simulink model "qless_forgetting_factor_16x16_nofifo"  (R2021a)
settings: Solver=FixedStepDiscrete  StartTime=0.0  StopTime=stoptime*inf  RelTol=1e-3
InitFcn:
  | qless_init_16chan_fi
undefined symbols (not defined in the file): fc, numArrayElements, physconst, srcAngles, Ts
libraries: hdlsllib x137, commfilt2 x4, commrfcorlib x3, commsync2 x3, commrflib2 x2, commrandsrc3 x2, simulink x2, phasedtxrxlib x2, commdigbbndcpm2 x1, embreciprocals x1, commdigbbndpm3 x1
(part 1 of 22)
Description:
  | MVDR HDL 4x4 systolic testbench
settings Model: DataTypeOverride=Off  SimulationMode=accelerator  Creator=The MathWorks, Inc.  LastModifiedBy=darenlee
settings SolverCC: AlgebraicLoopSolver=TrustRegion
settings DataIOCC: LimitDataPoints=on  SaveFormat=Array  SaveOutput=off  SaveTime=off  ReturnWorkspaceOutputs=off
settings OptimizationCC: BlockReduction=off  ConditionallyExecuteInputs=off  DefaultParameterBehavior=Inlined  LifeSpan=inf
settings DebuggingCC: ReadBeforeWriteMsg=DisableAll  WriteAfterWriteMsg=DisableAll  WriteAfterReadMsg=DisableAll  AlgebraicLoopMsg=error  UnderspecifiedInitializationDetection=Classic  MergeDetectMultiDrivingBlocksExec=none  SolverPrmCheckMsg=warning  SingleTaskRateTransMsg=error  ParameterPrecisionLossMsg=none  AllowSymbolicDim=off  SFUnexpectedBacktrackingDiag=warning  SFNoUnconditionalDefaultTransitionDiag=warning  SFExecutionAtInitializationDiag=none  SFMachineParentedDataDiag=warning  ArithmeticOperatorsInVariantConditions=warning
settings HardwareCC: ProdBitPerPointer=32  ProdBitPerSizeT=32  ProdBitPerPtrDiffT=32  ProdLargestAtomicFloat=None  ProdIntDivRoundTo=Undefined  ProdEndianess=Unspecified  ProdWordSize=32  ProdHWDeviceType=ASIC/FPGA->ASIC/FPGA  TargetBitPerPointer=64  TargetBitPerSizeT=64  TargetBitPerPtrDiffT=64  TargetLongLongMode=on  TargetIntDivRoundTo=Zero  TargetEndianess=LittleEndian  TargetWordSize=64  TargetHWDeviceType=Custom Processor->MATLAB Host Computer  ProdEqTarget=off
settings ModelReferenceCC: PropagateSignalLabelsOutOfModel=off
settings SFSimCC: SimUseLocalCustomCode=off  CustomCodeUndefinedFunction=UseInterfaceOnly
settings RTWCC: RTWUseLocalCustomCode=off
settings CodeAppCC: StateflowObjectComments=on
settings GRTTargetCC: TargetLangStandard=C89/C90 (ANSI)
settings ConfigComp: CovMetricSettings=dw  CovSaveCumulativeToWorkspaceVar=on  CovSaveSingleToWorkspaceVar=on  CovExternalEMLEnable=off  CovSFcnEnable=off

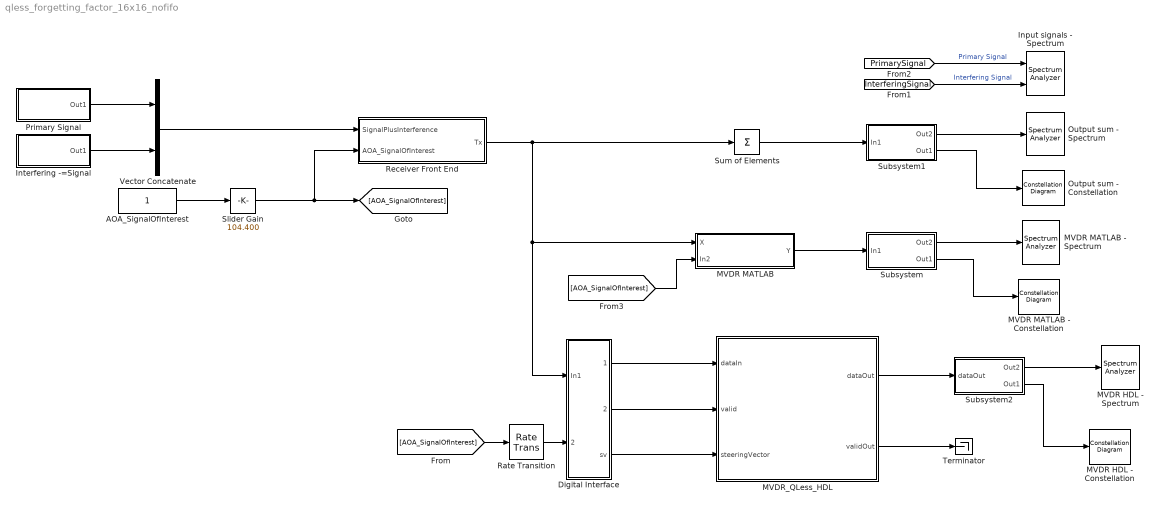
== system qless_forgetting_factor_16x16_nofifo ==
  AOA_SignalOfInterest : Constant  SampleTime=-1
  Digital Interface : Subsystem
  Input signals - Spectrum : SpectrumAnalyzer  NumInputPorts=2
  Interfering -=Signal : Subsystem
      mask Display: disp('Interfering\nSignal')
  MVDR HDL - Constellation : ConstellationDiagram
  MVDR HDL - Spectrum : SpectrumAnalyzer
  MVDR MATLAB : Subsystem
  MVDR MATLAB - Constellation : ConstellationDiagram
  MVDR MATLAB - Spectrum : SpectrumAnalyzer
  MVDR_QLess_HDL : Subsystem
  Output sum - Constellation : ConstellationDiagram
  Output sum - Spectrum : SpectrumAnalyzer
  Primary Signal : Subsystem
      mask Display: disp('Primary\nSignal')
  Rate Transition : RateTransition
  Receiver Front End : Subsystem
  Slider Gain : simulink/Math Operations/Slider Gain  gain=104.400  low=0  high=120
  Subsystem : Subsystem
  Subsystem1 : Subsystem
  Subsystem2 : Subsystem
  Sum of Elements : Sum  Inputs=+  CollapseMode=Specified dimension  CollapseDim=2
  Terminator : Terminator
  Vector Concatenate : Concatenate  Mode=Multidimensional array  ConcatenateDimension=2
  wires:
  MVDR MATLAB/1(Y) -> Subsystem/1(In1)
  Interfering -=Signal/1(Out1) -> Vector Concatenate/2
  Primary Signal/1(Out1) -> Vector Concatenate/1
  [InterferingSignal] -> Input signals - Spectrum/2  "Interfering Signal"
  Subsystem/2(Out1) -> MVDR MATLAB - Constellation/1
  Subsystem/1(Out2) -> MVDR MATLAB - Spectrum/1
  Sum of Elements/1 -> Subsystem1/1(In1)
  Subsystem1/1(Out2) -> Output sum - Spectrum/1
  Subsystem1/2(Out1) -> Output sum - Constellation/1
  Subsystem2/1(Out2) -> MVDR HDL - Spectrum/1
  Subsystem2/2(Out1) -> MVDR HDL - Constellation/1
  [PrimarySignal] -> Input signals - Spectrum/1  "Primary Signal"
  Digital Interface/1(data) -> MVDR_QLess_HDL/1(dataIn)
  Receiver Front End/1(Tx) -> Sum of Elements/1, Digital Interface/1(In1), MVDR MATLAB/1(X)
  Vector Concatenate/1 -> Receiver Front End/1(SignalPlusInterference)
  Digital Interface/3(sv) -> MVDR_QLess_HDL/3(steeringVector)
  Digital Interface/2(valid) -> MVDR_QLess_HDL/2(valid)
  MVDR_QLess_HDL/1(dataOut) -> Subsystem2/1(dataOut)
  AOA_SignalOfInterest/1 -> Slider Gain/1
  [AOA_SignalOfInterest] -> Rate Transition/1
  Rate Transition/1 -> Digital Interface/2(SteeringAngle)
  MVDR_QLess_HDL/2(validOut) -> Terminator/1
  [AOA_SignalOfInterest] -> MVDR MATLAB/2(In2)
  Slider Gain/1 -> [AOA_SignalOfInterest], Receiver Front End/2(AOA_SignalOfInterest)

== system qless_forgetting_factor_16x16_nofifo/Digital Interface ==
  In1 : Inport
  SteeringAngle : Inport  Port=2
  Constant : Constant  Value=fc  SampleTime=-1
  Constant1 : Constant  Value=true  SampleTime=-1
  Data Type Conversion : DataTypeConversion  OutDataTypeStr=sv_dt
  Delay : Delay  DelayLength=120
  Delay1 : Delay  DelayLength=120
  Input DTC : Subsystem
  MATLAB System : MATLABSystem  System=phased.SteeringVector  PropagationSpeed=physconst( 'LightSpeed' )  IncludeElementResponse=off  NumPhaseShifterBits=0  EnablePolarization=off  SimulateUsing=Code generation  SensorArray=sensorArray
      mask Type: phased.SteeringVector
      mask Display:
      | disp(['Steering' char(10) 'Vector']);
      | port_label('input',1,'Freq');
      | port_label('input',2,'Ang');
  Unbuffer : Unbuffer
  data : Outport
  valid : Outport  Port=2
  sv : Outport  Port=3
  wires:
  Unbuffer/1 -> Input DTC/1(In1)
  In1/1 -> Unbuffer/1
  Data Type Conversion/1 -> sv/1
  Constant1/1 -> Delay/1
  Input DTC/1(Out1) -> Delay1/1
  Constant/1 -> MATLAB System/1
  SteeringAngle/1 -> MATLAB System/2
  MATLAB System/1 -> Data Type Conversion/1
  Delay/1 -> valid/1
  Delay1/1 -> data/1

== system qless_forgetting_factor_16x16_nofifo/Interfering -=Signal ==
  GMSK Modulator Baseband : commdigbbndcpm2/GMSK Modulator Baseband  inputType=Bit  BT=.3  pulseLength=4  preHistory=1  phaseOffset=0  samplesPerSymbol=8  RateOptions=Enforce single-rate processing  outDataType=double
      settings: SourceProductBaseCode=CM
  Gain : Gain  Gain=1/40
  Memoryless Nonlinearity2 : commrflib2/Memoryless Nonlinearity  model_select=Cubic polynomial  linGaindB=39  GindB=0  iip3=43  am2pm=.8  LPwrLimAMPM=-2.5  UPwrLimAMPM=17.5  amam=[2.1587 1.1517]  ampm=[4.0033 9.1040]  x=[8.1081 1.5413 6.5202 -0.0718]  y=[4.6645 2.0965 10.88 -0.003]  p=0.5  GoutdB=0  vsat=1
      settings: SourceProductBaseCode=CM
  Random Integer Generator1 : commrandsrc3/Random Integer Generator  SetSize=2  SeedSource=Auto  Seed=0  SampleTime=4*Ts  SamplesPerFrame=100  OutputDataType=boolean  SimulateUsing=Interpreted execution
  Out1 : Outport  VectorParamsAs1DForOutWhenUnconnected=off
  tag scope: InterferingSignal=global
  wires:
  Memoryless Nonlinearity2/1 -> Gain/1
  GMSK Modulator Baseband/1 -> Memoryless Nonlinearity2/1
  Random Integer Generator1/1 -> GMSK Modulator Baseband/1
  Gain/1 -> Out1/1, [InterferingSignal]

== system qless_forgetting_factor_16x16_nofifo/MVDR MATLAB ==
  X : Inport
  In2 : Inport  Port=2
  Constant : Constant  Value=fc  SampleTime=-1
  MATLAB Function : MATLAB Function  TreatAsAtomicUnit=on
  MATLAB System : MATLABSystem  System=phased.SteeringVector  PropagationSpeed=physconst( 'LightSpeed' )  IncludeElementResponse=off  NumPhaseShifterBits=0  EnablePolarization=off  SimulateUsing=Code generation  SensorArray=sensorArray
      mask Type: phased.SteeringVector
      mask Display:
      | disp(['Steering' char(10) 'Vector']);
      | port_label('input',1,'Freq');
      | port_label('input',2,'Ang');
  Y : Outport
  wires:
  MATLAB Function/1(Y) -> Y/1
  X/1 -> MATLAB Function/1(X)
  In2/1 -> MATLAB System/2
  Constant/1 -> MATLAB System/1
  MATLAB System/1 -> MATLAB Function/2(sv)

== system qless_forgetting_factor_16x16_nofifo/MVDR_QLess_HDL ==
  dataIn : Inport
  valid : Inport  Port=2
  steeringVector : Inport  Port=3
  Complex Partial-Systolic Matrix Solve Using Q-less QR Decomposition with Forgetting Factor Manually Tiled n=16 : Subsystem  mask(Complex Partial-Systolic Matrix Solve Using Q-less QR Decomposition with Forgetting Factor){n=16, p=1, forgettingFactor=0.9983, OutputType=fixdt(1,24,11)}
      mask prompts: n "fixed:emblib:ColumnsInARowsInB"; p "fixed:emblib:ColumnsInB"; forgettingFactor "fixed:emblib:ForgettingFactor"; OutputType "fixed:emblib:OutputPrototype"
      mask help: fixed:help:ComplexPartialSystolicQlessQRMatrixSolveWithForgettingFactorDescription
      mask Help: eval('embblk.embhelp(gcb)')
      mask DialogControl n Prompt: Number of columns in matrix A and rows in matrix B
      mask DialogControl p Prompt: Number of columns in matrix B
      mask DialogControl forgettingFactor Prompt: Forgetting factor
      mask DialogControl OutputType Prompt: Output datatype
  Conjugate : Math  Operator=conj  SignedPower=on  RndMeth=Zero  SaturateOnIntegerOverflow=on
  Constant1 : Constant  Value=false  SampleTime=-1
  Data Type Conversion1 : DataTypeConversion  OutDataTypeStr=matrixdivin_dt
  Data Type Conversion2 : DataTypeConversion  OutDataTypeStr=fixdt(1,19,14)
  Delay : Delay  DelayLength=1
  Delay1 : Delay  DelayLength=1
  Detect Increase : simulink/Logic and Bit Operations/Detect Increase  vinit=0.0  OutDataTypeStr=boolean
  Form Beam : Subsystem
  From Data Bus : Subsystem
  Normalize Response : Subsystem
  Reshape : Reshape
  Terminator : Terminator
  To Data Bus : Subsystem
  Unit Delay Enabled Synchronous1 : hdlsllib/Discrete/Unit Delay Enabled Synchronous  InitialCondition=0  SampleTime=-1
      settings: SourceProductBaseCode=SL
  Unit Delay Enabled Synchronous2 : hdlsllib/Discrete/Unit Delay Enabled Synchronous  InitialCondition=0  SampleTime=-1
      settings: SourceProductBaseCode=SL
  Unit Delay Enabled Synchronous3 : hdlsllib/Discrete/Unit Delay Enabled Synchronous  InitialCondition=0  SampleTime=-1
      settings: SourceProductBaseCode=SL
  dataOut : Outport
  validOut : Outport  Port=2
  wires:
  dataIn/1 -> Reshape/1, To Data Bus/1(data)
  Reshape/1 -> Unit Delay Enabled Synchronous1/1
  steeringVector/1 -> [sv]
  Delay/1 -> Complex Partial-Systolic Matrix Solve Using Q-less QR Decomposition with Forgetting Factor Manually Tiled n=16/3(validInA), Complex Partial-Systolic Matrix Solve Using Q-less QR Decomposition with Forgetting Factor Manually Tiled n=16/4(validInB)  "A_valid"
  Unit Delay Enabled Synchronous1/1 -> Data Type Conversion1/1
  Unit Delay Enabled Synchronous3/1 -> Data Type Conversion2/1
  From Data Bus/2(valid) -> Form Beam/2(validIn)
  From Data Bus/1(data) -> Form Beam/1(dataIn)
  Normalize Response/1(wOut) -> Form Beam/3(w)
  [sv] -> Normalize Response/3(steeringVector)
  To Data Bus/1(bus) -> From Data Bus/1(bus)
  Form Beam/1(dataOut) -> dataOut/1
  Form Beam/2(validOut) -> validOut/1
  Delay1/1 -> Normalize Response/2(validIn)
  Unit Delay Enabled Synchronous2/1 -> Normalize Response/1(wIn)
  Data Type Conversion1/1 -> Conjugate/1
  Data Type Conversion2/1 -> Complex Partial-Systolic Matrix Solve Using Q-less QR Decomposition with Forgetting Factor Manually Tiled n=16/2(B)
  Conjugate/1 -> Complex Partial-Systolic Matrix Solve Using Q-less QR Decomposition with Forgetting Factor Manually Tiled n=16/1(A(i,:))  "A_in"
  Constant1/1 -> Complex Partial-Systolic Matrix Solve Using Q-less QR Decomposition with Forgetting Factor Manually Tiled n=16/5(restart)
  Complex Partial-Systolic Matrix Solve Using Q-less QR Decomposition with Forgetting Factor Manually Tiled n=16/3(readyA) -> Detect Increase/1  "qr_rdy"
  Complex Partial-Systolic Matrix Solve Using Q-less QR Decomposition with Forgetting Factor Manually Tiled n=16/1(X) -> Unit Delay Enabled Synchronous2/1  "X"
  Complex Partial-Systolic Matrix Solve Using Q-less QR Decomposition with Forgetting Factor Manually Tiled n=16/2(validOut) -> Delay1/1, Unit Delay Enabled Synchronous2/2  "X_valid"
  [sv] -> Unit Delay Enabled Synchronous3/1
  Complex Partial-Systolic Matrix Solve Using Q-less QR Decomposition with Forgetting Factor Manually Tiled n=16/4(readyB) -> Terminator/1
  Detect Increase/1 -> Unit Delay Enabled Synchronous1/2, Unit Delay Enabled Synchronous3/2, Delay/1
  valid/1 -> To Data Bus/2(valid)

== system qless_forgetting_factor_16x16_nofifo/Primary Signal ==
  Gain : Gain  Gain=1/40
  Memoryless Nonlinearity : commrflib2/Memoryless Nonlinearity  model_select=Cubic polynomial  linGaindB=28  GindB=0  iip3=43  am2pm=.8  LPwrLimAMPM=-2.5  UPwrLimAMPM=17.5  amam=[2.1587 1.1517]  ampm=[4.0033 9.1040]  x=[8.1081 1.5413 6.5202 -0.0718]  y=[4.6645 2.0965 10.88 -0.003]  p=0.5  GoutdB=0  vsat=1
      settings: SourceProductBaseCode=CM
  QPSK Modulator Baseband : commdigbbndpm3/QPSK Modulator Baseband  InType=Integer  Enc=Gray  Ph=pi/4  outDtype=double  outWordLen=16  outUDDataType=sfix(16)  outFracLenMode=Best precision  outFracLen=15  outDataTypeStr=double  outLastDataTypeStr=double
  Raised Cosine Transmit Filter : commfilt2/Raised Cosine Transmit Filter  filtType=Square root  R=.3  filtSpan=10  N=2  filterGain=1  InputProcessing=Columns as channels (frame based)  RateOptions=Enforce single-rate processing  framing=Mute  checkCoeff=off  variableName=rcTxFilt  checkGain=Normalized  sampMode=Mute  saveAsFlag=0  currentFiltSpan=10  D=(10)/2  launchFVT=on  roundingMode=Floor  overflowMode=off  coeffDataTypeStr=Inherit: Same word length as input  coeffMin=[]  coeffMax=[]  coeffLastDataTypeStr=Inherit: Same word length as input  outputDataTypeStr=Inherit: Same as accumulator  outputMin=[]  outputMax=[]  outputLastDataTypeStr=Inherit: Same as accumulator
  Random Integer Generator : commrandsrc3/Random Integer Generator  SetSize=4  SeedSource=Auto  Seed=0  SampleTime=Ts  SamplesPerFrame=400  OutputDataType=double  SimulateUsing=Interpreted execution
  Out1 : Outport  VectorParamsAs1DForOutWhenUnconnected=off
  tag scope: PrimarySignal=global
  wires:
  QPSK Modulator Baseband/1 -> Raised Cosine Transmit Filter/1
  Random Integer Generator/1 -> QPSK Modulator Baseband/1
  Memoryless Nonlinearity/1 -> Gain/1
  Raised Cosine Transmit Filter/1 -> Memoryless Nonlinearity/1
  Gain/1 -> Out1/1, [PrimarySignal]

== system qless_forgetting_factor_16x16_nofifo/Receiver Front End ==
  SignalPlusInterference : Inport
  AOA_SignalOfInterest : Inport  Port=2
  Constant1 : Constant  Value=srcAngles(2)  SampleTime=-1
  Narrowband Receive Array : phasedtxrxlib/Narrowband Receive Array  PropagationSpeed=propSpeed  OperatingFrequency=fc  Wavefront=Plane  SensorGainMeasure=dB  Polarization=None  WeightsInputPort=off  SimulateUsing=Interpreted execution  Sensor=sensorArray
      settings: SourceProductBaseCode=AR
  Receiver Preamp : phasedtxrxlib/Receiver Preamp  Gain=-10  LossFactor=0  NoiseMethod=Noise power  NoiseFigure=0  ReferenceTemperature=290  SampleRateFromInputCheckbox=on  SampleRate=1e6  NoisePower=.001  EnableInputPort=off  PhaseNoiseInputPort=off  SeedSource=Auto  Seed=0  SimulateUsing=Interpreted execution
      settings: SourceProductBaseCode=AR
  Reshape : Reshape  OutputDimensionality=Row vector (2-D)
  Vector Concatenate : Concatenate
  Tx : Outport
  wires:
  SignalPlusInterference/1 -> Narrowband Receive Array/1
  Narrowband Receive Array/1 -> Receiver Preamp/1
  Reshape/1 -> Narrowband Receive Array/2
  Receiver Preamp/1 -> Tx/1
  Vector Concatenate/1 -> Reshape/1
  AOA_SignalOfInterest/1 -> Vector Concatenate/1
  Constant1/1 -> Vector Concatenate/2

== system qless_forgetting_factor_16x16_nofifo/Subsystem ==
  In1 : Inport
  AGC : commrfcorlib/AGC  LegacyMode=off  DetectorMethod=Rectifier  LoopMethod=Linear  UpdatePeriod=100  StepSize=0.1  AdaptationStepSize=0.01  DesiredOutputPower=1  AveragingLength=200  MaximumGain=30  MaxPowerGain=60  GainOutputPort=off  InputPowerOutputPort=off  SimulateUsing=Interpreted execution
  Carrier Synchronizer : commsync2/Carrier Synchronizer  Modulation=QPSK  ModulationPhaseOffset=Auto  CustomPhaseOffset=0  SamplesPerSymbol=1  DampingFactor=0.707  NormalizedLoopBandwidth=0.01  EstimatedPhaseErrorOutputPort=off  SimulateUsing=Interpreted execution
  Raised Cosine Receive Filter : commfilt2/Raised Cosine Receive Filter  filtType=Square root  R=.3  filtSpan=10  N=2  downFactor=2  downOffset=0  filterGain=1  InputProcessing=Columns as channels (frame based)  RateOptions=Enforce single-rate processing  framing=Mute  checkCoeff=off  variableName=rcRxFilt  currentFiltSpan=10  D=5  inputOffset=0  sampMode=Mute  saveAsFlag=0  rateMode=Downsampling  checkGain=Normalized  launchFVT=on  roundingMode=Floor  overflowMode=off  coeffDataTypeStr=Inherit: Same word length as input  coeffMin=[]  coeffMax=[]  coeffLastDataTypeStr=Inherit: Same word length as input  accumDataTypeStr=Inherit: Same as product output  accumLastDataTypeStr=Inherit: Same as product output  outputDataTypeStr=Inherit: Same as accumulator  outputMin=[]  outputMax=[]  outputLastDataTypeStr=Inherit: Same as accumulator
  Out2 : Outport
  Out1 : Outport  Port=2
  wires:
  In1/1 -> Out2/1, Raised Cosine Receive Filter/1
  Raised Cosine Receive Filter/1 -> Carrier Synchronizer/1
  AGC/1 -> Out1/1
  Carrier Synchronizer/1 -> AGC/1

== system qless_forgetting_factor_16x16_nofifo/Subsystem1 ==
  In1 : Inport
  AGC : commrfcorlib/AGC  LegacyMode=off  DetectorMethod=Rectifier  LoopMethod=Linear  UpdatePeriod=100  StepSize=0.1  AdaptationStepSize=0.01  DesiredOutputPower=1  AveragingLength=200  MaximumGain=30  MaxPowerGain=60  GainOutputPort=off  InputPowerOutputPort=off  SimulateUsing=Interpreted execution
  Carrier Synchronizer : commsync2/Carrier Synchronizer  Modulation=QPSK  ModulationPhaseOffset=Auto  CustomPhaseOffset=0  SamplesPerSymbol=1  DampingFactor=0.707  NormalizedLoopBandwidth=0.01  EstimatedPhaseErrorOutputPort=off  SimulateUsing=Interpreted execution
  Raised Cosine Receive Filter : commfilt2/Raised Cosine Receive Filter  filtType=Square root  R=.3  filtSpan=10  N=2  downFactor=2  downOffset=0  filterGain=1  InputProcessing=Columns as channels (frame based)  RateOptions=Enforce single-rate processing  framing=Mute  checkCoeff=off  variableName=rcRxFilt  currentFiltSpan=10  D=5  inputOffset=0  sampMode=Mute  saveAsFlag=0  rateMode=Downsampling  checkGain=Normalized  launchFVT=on  roundingMode=Floor  overflowMode=off  coeffDataTypeStr=Inherit: Same word length as input  coeffMin=[]  coeffMax=[]  coeffLastDataTypeStr=Inherit: Same word length as input  accumDataTypeStr=Inherit: Same as product output  accumLastDataTypeStr=Inherit: Same as product output  outputDataTypeStr=Inherit: Same as accumulator  outputMin=[]  outputMax=[]  outputLastDataTypeStr=Inherit: Same as accumulator
  Out2 : Outport
  Out1 : Outport  Port=2
  wires:
  Carrier Synchronizer/1 -> AGC/1
  AGC/1 -> Out1/1
  Raised Cosine Receive Filter/1 -> Carrier Synchronizer/1
  In1/1 -> Raised Cosine Receive Filter/1, Out2/1

== system qless_forgetting_factor_16x16_nofifo/Subsystem2 ==
  dataOut : Inport
  AGC : commrfcorlib/AGC  LegacyMode=off  DetectorMethod=Rectifier  LoopMethod=Linear  UpdatePeriod=100  StepSize=0.1  AdaptationStepSize=0.01  DesiredOutputPower=1  AveragingLength=200  MaximumGain=30  MaxPowerGain=60  GainOutputPort=off  InputPowerOutputPort=off  SimulateUsing=Interpreted execution
  Buffer : Buffer  N=800  OutputFrames=off
  Carrier Synchronizer : commsync2/Carrier Synchronizer  Modulation=QPSK  ModulationPhaseOffset=Auto  CustomPhaseOffset=0  SamplesPerSymbol=1  DampingFactor=0.707  NormalizedLoopBandwidth=0.01  EstimatedPhaseErrorOutputPort=off  SimulateUsing=Interpreted execution
  Data Type Conversion : DataTypeConversion  OutDataTypeStr=double
  Raised Cosine Receive Filter : commfilt2/Raised Cosine Receive Filter  filtType=Square root  R=.3  filtSpan=10  N=2  downFactor=2  downOffset=0  filterGain=1  InputProcessing=Columns as channels (frame based)  RateOptions=Enforce single-rate processing  framing=Mute  checkCoeff=off  variableName=rcRxFilt  currentFiltSpan=10  D=5  inputOffset=0  sampMode=Mute  saveAsFlag=0  rateMode=Downsampling  checkGain=Normalized  launchFVT=on  roundingMode=Floor  overflowMode=off  coeffDataTypeStr=Inherit: Same word length as input  coeffMin=[]  coeffMax=[]  coeffLastDataTypeStr=Inherit: Same word length as input  accumDataTypeStr=Inherit: Same as product output  accumLastDataTypeStr=Inherit: Same as product output  outputDataTypeStr=Inherit: Same as accumulator  outputMin=[]  outputMax=[]  outputLastDataTypeStr=Inherit: Same as accumulator
  Out2 : Outport
  Out1 : Outport  Port=2
  wires:
  Carrier Synchronizer/1 -> AGC/1
  AGC/1 -> Out1/1
  Raised Cosine Receive Filter/1 -> Carrier Synchronizer/1
  dataOut/1 -> Buffer/1
  Buffer/1 -> Data Type Conversion/1
  Data Type Conversion/1 -> Raised Cosine Receive Filter/1, Out2/1

== system qless_forgetting_factor_16x16_nofifo/Digital Interface/Input DTC ==
  In1 : Inport
  Data Type Conversion : DataTypeConversion  OutDataTypeStr=input_dt
  Data Type Conversion1 : DataTypeConversion  OutDataTypeStr=adc_dt
  Out1 : Outport
  wires:
  Data Type Conversion/1 -> Out1/1
  In1/1 -> Data Type Conversion1/1
  Data Type Conversion1/1 -> Data Type Conversion/1

== system qless_forgetting_factor_16x16_nofifo/MVDR_QLess_HDL/Complex Partial-Systolic Matrix Solve Using Q-less QR Decomposition with Forgetting Factor Manually Tiled n=16 ==
  A(i,:) : Inport
  B : Inport  Port=2
  validInA : Inport  Port=3
  validInB : Inport  Port=4
  restart : Inport  Port=5
  Complex Partial-Systolic Q-less QR with Forgetting Factor : Subsystem  mask(Complex Partial-Systolic Q-less QR with Forgetting Factor){n=16, forgettingFactor=forgettingFactor}
      mask prompts: n "fixed:emblib:ColumnsInA"; forgettingFactor "fixed:emblib:ForgettingFactor"
      mask help: fixed:help:ComplexPartialSystolicQlessQRwithForgettingFactorDescription
      mask init:
      | embblk.burstqr.checkHDLInOutPipeline(gcb);
      mask Help: eval('embblk.embhelp(gcb)')
      mask DialogControl n Prompt: Number of columns in matrix A
      mask DialogControl forgettingFactor Prompt: Forgetting factor
  Complex Q-less QR Forward Backward Substitute : Subsystem  mask(Complex Q-less QR Forward Backward Substitute){n=n, p=p, OutputType=OutputType}
      mask prompts: n "fixed:emblib:ColumnsInARowsInB"; p "fixed:emblib:ColumnsInB"; OutputType "fixed:emblib:OutputPrototype"
      mask help: fixed:help:ComplexForwardBackwardSubstituteDescription
      mask Help: fixed:emblib:InternalUseOnly
      mask DialogControl n Prompt: Number of columns in matrix A and rows in matrix B
      mask DialogControl p Prompt: Number of columns in matrix B
      mask DialogControl OutputType Prompt: Output datatype
  Delay : Delay  DelayLength=1
  Unit Delay Enabled Synchronous : hdlsllib/Discrete/Unit Delay Enabled Synchronous  InitialCondition=0.0  SampleTime=-1
      settings: SourceProductBaseCode=SL
  X : Outport
  validOut : Outport  Port=2
  readyA : Outport  Port=3
  readyB : Outport  Port=4
  wires:
  validInB/1 -> Complex Q-less QR Forward Backward Substitute/4(validInB)
  B/1 -> Complex Q-less QR Forward Backward Substitute/2(B)
  Complex Q-less QR Forward Backward Substitute/3(ready) -> readyB/1
  Unit Delay Enabled Synchronous/1 -> Complex Q-less QR Forward Backward Substitute/1(R)
  Delay/1 -> Complex Q-less QR Forward Backward Substitute/3(validInR)
  Complex Q-less QR Forward Backward Substitute/2(validOut) -> validOut/1
  Complex Q-less QR Forward Backward Substitute/1(X) -> X/1
  Complex Partial-Systolic Q-less QR with Forgetting Factor/2(validOut) -> Unit Delay Enabled Synchronous/2, Delay/1
  Complex Partial-Systolic Q-less QR with Forgetting Factor/3(ready) -> readyA/1
  validInA/1 -> Complex Partial-Systolic Q-less QR with Forgetting Factor/2(validIn)
  restart/1 -> Complex Partial-Systolic Q-less QR with Forgetting Factor/3(restart), Complex Q-less QR Forward Backward Substitute/5(restart)
  Complex Partial-Systolic Q-less QR with Forgetting Factor/1(R) -> Unit Delay Enabled Synchronous/1
  A(i,:)/1 -> Complex Partial-Systolic Q-less QR with Forgetting Factor/1(A(i,:))

== system qless_forgetting_factor_16x16_nofifo/MVDR_QLess_HDL/Form Beam ==
  dataIn : Inport
  validIn : Inport  Port=2
  w : Inport  Port=3
  Data Type Conversion : DataTypeConversion  OutDataTypeStr=output_dt
  Delay1 : Delay  DelayLength=6
  Delay2 : Delay
  Math Function2 : Math  Operator=conj  SaturateOnIntegerOverflow=on
  Parallel Complex Multiply : Subsystem  TreatAsAtomicUnit=on
  Reshape : Reshape
  Reshape1 : Reshape
  Tree Sum : Subsystem
  dataOut : Outport
  validOut : Outport  Port=2
  wires:
  dataIn/1 -> Reshape1/1
  Parallel Complex Multiply/1(z) -> Tree Sum/1(In1)
  Tree Sum/1(Out1) -> Data Type Conversion/1
  Math Function2/1 -> Reshape/1
  w/1 -> Math Function2/1
  validIn/1 -> Delay1/1
  Reshape/1 -> Parallel Complex Multiply/2(z2)
  Reshape1/1 -> Parallel Complex Multiply/1(z1)
  Data Type Conversion/1 -> dataOut/1
  Delay2/1 -> validOut/1
  Delay1/1 -> Delay2/1

== system qless_forgetting_factor_16x16_nofifo/MVDR_QLess_HDL/From Data Bus ==
  bus : Inport
  Bus Selector : BusSelector  OutputSignals=data,valid
  data : Outport
  valid : Outport  Port=2
  wires:
  Bus Selector/2 -> valid/1  "<valid>"
  Bus Selector/1 -> data/1  "<data>"
  bus/1 -> Bus Selector/1

== system qless_forgetting_factor_16x16_nofifo/MVDR_QLess_HDL/Normalize Response ==
  note: This subsystem scales the weight vector to ensure unit gain in the target direction.
  wIn : Inport
  validIn : Inport  Port=2
  steeringVector : Inport  Port=3
  MVDR Weight Update : Subsystem
  Unit Delay Enabled Synchronous : hdlsllib/Discrete/Unit Delay Enabled Synchronous  InitialCondition=0.0  SampleTime=-1
      settings: SourceProductBaseCode=SL
  wOut : Outport
  wires:
  steeringVector/1 -> MVDR Weight Update/1(Steering Vector)
  wIn/1 -> MVDR Weight Update/2(x)
  MVDR Weight Update/1(w) -> Unit Delay Enabled Synchronous/1
  MVDR Weight Update/2(validOut) -> Unit Delay Enabled Synchronous/2
  Unit Delay Enabled Synchronous/1 -> wOut/1
  validIn/1 -> MVDR Weight Update/3(validIn)

== system qless_forgetting_factor_16x16_nofifo/MVDR_QLess_HDL/To Data Bus ==
  data : Inport
  valid : Inport  Port=2
  Bus Creator : BusCreator  Inputs=2
  bus : Outport
  wires:
  data/1 -> Bus Creator/1  "data"
  Bus Creator/1 -> bus/1
  valid/1 -> Bus Creator/2  "valid"

== system qless_forgetting_factor_16x16_nofifo/MVDR_QLess_HDL/Complex Partial-Systolic Matrix Solve Using Q-less QR Decomposition with Forgetting Factor Manually Tiled n=16/Complex Partial-Systolic Q-less QR with Forgetting Factor ==
  A(i,:) : Inport
  validIn : Inport  Port=2
  restart : Inport  Port=3
  Complex Partial-Systolic Q-less QR with Forgetting Factor Manually tiled : Subsystem  TreatAsAtomicUnit=on  mask{n=16, forgettingFactor=forgettingFactor}
      mask prompts: n "fixed:emblib:ColumnsInA"; forgettingFactor "fixed:emblib:ForgettingFactor"
      mask DialogControl n Prompt: Number of columns in matrix A
      mask DialogControl forgettingFactor Prompt: Forgetting factor
  Delay{,1..2,5..6} (5 alike) : Delay  DelayLength=1
  Partial-Systolic Q-less QR with Forgetting Factor Output Memory Manager : Subsystem  mask{n=n}
      mask prompts: n "fixed:emblib:ColumnsInA"
      mask DialogControl n Prompt: Number of columns in matrix A
      mask Display: disp('Partial-Systolic Q-less QR \nwith Forgetting Factor \nOutput Memory Manager')
  Reshape2 : Reshape  OutputDimensionality=Row vector (2-D)
  Reshape4 : Reshape  OutputDimensionality=Customize  OutputDimensions=[n,n]
  Transpose : Math  Operator=transpose  SaturateOnIntegerOverflow=on
  R : Outport
  validOut : Outport  Port=2
  ready : Outport  Port=3
  wires:
  Transpose/1 -> Delay5/1
  Delay5/1 -> R/1
  Partial-Systolic Q-less QR with Forgetting Factor Output Memory Manager/1(RtransposeOut) -> Reshape4/1
  Reshape4/1 -> Transpose/1
  Delay/1 -> Partial-Systolic Q-less QR with Forgetting Factor Output Memory Manager/1(RtransposeIn)
  Partial-Systolic Q-less QR with Forgetting Factor Output Memory Manager/2(validOut) -> Delay6/1
  Delay1/1 -> Partial-Systolic Q-less QR with Forgetting Factor Output Memory Manager/2(validIn)
  Complex Partial-Systolic Q-less QR with Forgetting Factor Manually tiled/1(R(i,:).') -> Delay/1
  Delay6/1 -> validOut/1
  A(i,:)/1 -> Reshape2/1
  restart/1 -> Partial-Systolic Q-less QR with Forgetting Factor Output Memory Manager/3(restart), Complex Partial-Systolic Q-less QR with Forgetting Factor Manually tiled/3(restart)
  Complex Partial-Systolic Q-less QR with Forgetting Factor Manually tiled/3(ready) -> Delay2/1
  validIn/1 -> Complex Partial-Systolic Q-less QR with Forgetting Factor Manually tiled/2(validIn)
  Reshape2/1 -> Complex Partial-Systolic Q-less QR with Forgetting Factor Manually tiled/1(A(i,:))
  Complex Partial-Systolic Q-less QR with Forgetting Factor Manually tiled/2(validR) -> Delay1/1
  Delay2/1 -> ready/1

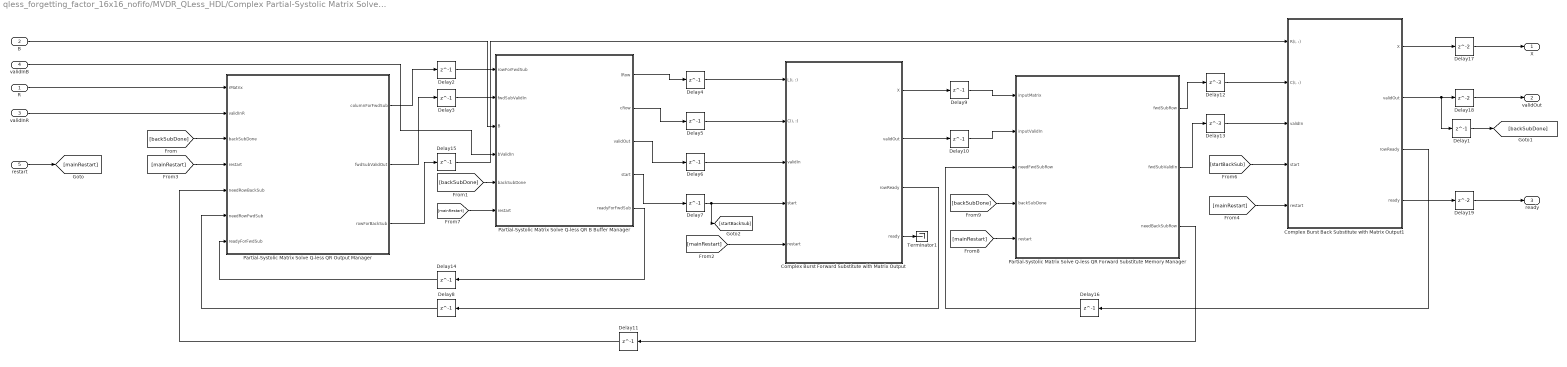
== system qless_forgetting_factor_16x16_nofifo/MVDR_QLess_HDL/Complex Partial-Systolic Matrix Solve Using Q-less QR Decomposition with Forgetting Factor Manually Tiled n=16/Complex Q-less QR Forward Backward Substitute ==
  R : Inport
  B : Inport  Port=2
  validInR : Inport  Port=3
  validInB : Inport  Port=4
  restart : Inport  Port=5
  Complex Burst Back Substitute with Matrix Output1 : Subsystem  mask(Complex Burst Back Substitute){n=n, p=p, OutputType=OutputType}
      mask prompts: n "fixed:emblib:ColumnsInA"; p "fixed:emblib:ColumnsInB"; OutputType "fixed:emblib:OutputPrototype"
      mask help: fixed:help:ComplexBackSubstituteDescription
      mask Help: fixed:emblib:InternalUseOnly
      mask DialogControl n Prompt: Number of columns in matrix A
      mask DialogControl p Prompt: Number of columns in matrix B
      mask DialogControl OutputType Prompt: Output datatype
  Complex Burst Forward Substitute with Matrix Output : Subsystem  mask(Complex Burst Forward Substitute){n=n, p=p, OutputType=OutputType}
      mask prompts: n "fixed:emblib:ColumnsInA"; p "fixed:emblib:ColumnsInB"; OutputType "fixed:emblib:OutputPrototype"
      mask help: fixed:emblib:ComplexForwardSubstituteDescription
      mask Help: fixed:emblib:InternalUseOnly
      mask DialogControl n Prompt: Number of columns in matrix A
      mask DialogControl p Prompt: Number of columns in matrix B
      mask DialogControl OutputType Prompt: Output datatype
  Delay{1..11,14..16} (14 alike) : Delay  DelayLength=1
  Delay12 : Delay  DelayLength=3
  Delay13 : Delay  DelayLength=3
  Delay17 : Delay
  Delay18 : Delay
  Delay19 : Delay
  Partial-Systolic Matrix Solve Q-less QR B Buffer Manager : Subsystem  mask{n=n, p=p}
      mask prompts: n "fixed:emblib:ColumnsInA"; p "fixed:emblib:ColumnsInB"
      mask DialogControl n Prompt: Number of columns in matrix A
      mask DialogControl p Prompt: Number of columns in matrix B
      mask Display: disp('Partial-Systolic Matrix Solve\nQ-less QR B Buffer Manager')
  Partial-Systolic Matrix Solve Q-less QR Forward Substitute Memory Manager : Subsystem  mask{n=n, p=p}
      mask prompts: n "fixed:emblib:ColumnsInA"; p "fixed:emblib:ColumnsInB"
      mask DialogControl n Prompt: Number of columns in matrix A
      mask DialogControl p Prompt: Number of columns in matrix B
      mask Display: disp('Partial-Systolic Matrix Solve\nQ-less QR\nForward Substitute Memory Manager')
  Partial-Systolic Matrix Solve Q-less QR Output Manager : Subsystem  mask{n=n}
      mask prompts: n "fixed:emblib:ColumnsInA"
      mask DialogControl n Prompt: Number of columns in matrix A
      mask Display: disp('Partial-Systolic Matrix Solve\nQ-less QR Output Manager')
  Terminator1 : Terminator
  X : Outport
  validOut : Outport  Port=2
  ready : Outport  Port=3
  wires:
  [mainRestart] -> Partial-Systolic Matrix Solve Q-less QR Output Manager/4(restart)
  [backSubDone] -> Partial-Systolic Matrix Solve Q-less QR Output Manager/3(backSubDone)
  Delay19/1 -> ready/1
  Delay18/1 -> validOut/1
  Delay17/1 -> X/1
  R/1 -> Partial-Systolic Matrix Solve Q-less QR Output Manager/1(rMatrix)
  Complex Burst Forward Substitute with Matrix Output/1(X) -> Delay9/1
  Delay4/1 -> Complex Burst Forward Substitute with Matrix Output/1("L(i, :)")
  Complex Burst Back Substitute with Matrix Output1/4(ready) -> Delay19/1
  Delay5/1 -> Complex Burst Forward Substitute with Matrix Output/2("C(i, :)")
  restart/1 -> [mainRestart]
  B/1 -> Partial-Systolic Matrix Solve Q-less QR B Buffer Manager/3(B)
  Delay15/1 -> Complex Burst Back Substitute with Matrix Output1/1("R(i, :)")
  Partial-Systolic Matrix Solve Q-less QR Forward Substitute Memory Manager/1(fwdSubRow) -> Delay12/1
  [mainRestart] -> Partial-Systolic Matrix Solve Q-less QR B Buffer Manager/6(restart)
  Delay9/1 -> Partial-Systolic Matrix Solve Q-less QR Forward Substitute Memory Manager/1(inputMatrix)
  Delay14/1 -> Partial-Systolic Matrix Solve Q-less QR Output Manager/7(readyForFwdSub)
  Complex Burst Back Substitute with Matrix Output1/2(validOut) -> Delay1/1, Delay18/1
  Delay7/1 -> Complex Burst Forward Substitute with Matrix Output/4(start), [startBackSub]
  Partial-Systolic Matrix Solve Q-less QR B Buffer Manager/4(start) -> Delay7/1
  validInB/1 -> Partial-Systolic Matrix Solve Q-less QR B Buffer Manager/4(bValidIn)
  Partial-Systolic Matrix Solve Q-less QR B Buffer Manager/3(validOut) -> Delay6/1
  Partial-Systolic Matrix Solve Q-less QR Forward Substitute Memory Manager/2(fwdSubValidIn) -> Delay13/1
  Partial-Systolic Matrix Solve Q-less QR B Buffer Manager/5(readyForFwdSub) -> Delay14/1
  Delay1/1 -> [backSubDone]
  Delay12/1 -> Complex Burst Back Substitute with Matrix Output1/2("C(i, :)")
  [mainRestart] -> Partial-Systolic Matrix Solve Q-less QR Forward Substitute Memory Manager/5(restart)
  Delay16/1 -> Partial-Systolic Matrix Solve Q-less QR Forward Substitute Memory Manager/3(needFwdSubRow)
  Complex Burst Forward Substitute with Matrix Output/4(ready) -> Terminator1/1
  [backSubDone] -> Partial-Systolic Matrix Solve Q-less QR B Buffer Manager/5(backSubDone)
  Delay6/1 -> Complex Burst Forward Substitute with Matrix Output/3(validIn)
  Partial-Systolic Matrix Solve Q-less QR Forward Substitute Memory Manager/3(needBackSubRow) -> Delay11/1
  Complex Burst Back Substitute with Matrix Output1/3(rowReady) -> Delay16/1
  Partial-Systolic Matrix Solve Q-less QR B Buffer Manager/2(cRow) -> Delay5/1
  Delay13/1 -> Complex Burst Back Substitute with Matrix Output1/3(validIn)
  Delay8/1 -> Partial-Systolic Matrix Solve Q-less QR Output Manager/6(needRowFwdSub)
  Complex Burst Back Substitute with Matrix Output1/1(X) -> Delay17/1
  Partial-Systolic Matrix Solve Q-less QR Output Manager/3(rowForBackSub) -> Delay15/1
  Delay2/1 -> Partial-Systolic Matrix Solve Q-less QR B Buffer Manager/1(rowForFwdSub)
  [backSubDone] -> Partial-Systolic Matrix Solve Q-less QR Forward Substitute Memory Manager/4(backSubDone)
  Complex Burst Forward Substitute with Matrix Output/3(rowReady) -> Delay8/1
  [startBackSub] -> Complex Burst Back Substitute with Matrix Output1/4(start)
  Partial-Systolic Matrix Solve Q-less QR B Buffer Manager/1(lRow) -> Delay4/1
  Delay10/1 -> Partial-Systolic Matrix Solve Q-less QR Forward Substitute Memory Manager/2(inputValidIn)
  Complex Burst Forward Substitute with Matrix Output/2(validOut) -> Delay10/1
  [mainRestart] -> Complex Burst Back Substitute with Matrix Output1/5(restart)
  Partial-Systolic Matrix Solve Q-less QR Output Manager/2(fwdSubValidOut) -> Delay3/1
  Partial-Systolic Matrix Solve Q-less QR Output Manager/1(columnForFwdSub) -> Delay2/1
  Delay11/1 -> Partial-Systolic Matrix Solve Q-less QR Output Manager/5(needRowBackSub)
  validInR/1 -> Partial-Systolic Matrix Solve Q-less QR Output Manager/2(validInR)
  [mainRestart] -> Complex Burst Forward Substitute with Matrix Output/5(restart)
  Delay3/1 -> Partial-Systolic Matrix Solve Q-less QR B Buffer Manager/2(fwdSubValidIn)

== system qless_forgetting_factor_16x16_nofifo/MVDR_QLess_HDL/Form Beam/Parallel Complex Multiply ==
  z1 : Inport  Partition=on  PartitionDimension=1  PartitionWidth=1  PartitionOffset=0
  z2 : Inport  Port=2  Partition=on  PartitionDimension=1  PartitionWidth=1  PartitionOffset=0
  For Each : ForEach  DisableCoverage=on
  HDL Complex Multiply : Subsystem  mask(HDL Complex Multiplier (3 Multiply, 5 Add)){D1=2, D2=1, D3=1, D4=1, D5=1}
      mask help:
      | Xilinx devices:
      | - Set D1 = 1 or 2 to trade off speed & FF resources
      | - Set D2-D5 = 1 to fully leverage DSP48 pipelines
      | - Use sync reset
      |
      | Intel FPGAs:
      | - Set D1 = 1 or 2 depending on device family
      | - Set D5 = 1; D2, D3, D4 = 0
      | - Use async reset
      mask init:
      | delay = D1+D2+D3+D4+D5;
      mask Display:
      | fprintf('Delay=%d',delay);
      | port_label('input',1,'z1');
      | port_label('input',2,'z2');
  z : Outport  ConcatenationDimension=1
  wires:
  z1/1 -> HDL Complex Multiply/1(In1)
  z2/1 -> HDL Complex Multiply/2(In2)
  HDL Complex Multiply/1(Out1) -> z/1

== system qless_forgetting_factor_16x16_nofifo/MVDR_QLess_HDL/Form Beam/Tree Sum ==
  In1 : Inport
  Delay3 : Delay  DelayLength=ceil(log2(numArrayElements))
  Tree Sum of Elements : Sum  Inputs=+  OutDataTypeStr=Inherit: Same as first input  LockScale=on
  Out1 : Outport
  wires:
  Delay3/1 -> Out1/1
  In1/1 -> Tree Sum of Elements/1
  Tree Sum of Elements/1 -> Delay3/1

== system qless_forgetting_factor_16x16_nofifo/MVDR_QLess_HDL/Normalize Response/MVDR Weight Update ==
  Steering Vector : Inport
  x : Inport  Port=2
  validIn : Inport  Port=3
  Delay{,1,3..6} (6 alike) : Delay  DelayLength=1
  Delay2 : Delay  DelayLength=8
  Inner Product : Subsystem
  Vector / Scalar Divide : Subsystem
  w : Outport
  validOut : Outport  Port=2
  wires:
  x/1 -> Delay3/1
  Vector / Scalar Divide/1(w) -> w/1
  Delay4/1 -> Inner Product/1(u)
  Inner Product/1(y) -> Delay5/1
  Delay6/1 -> Vector / Scalar Divide/1(x)
  Delay/1 -> Vector / Scalar Divide/3(validIn)
  Steering Vector/1 -> Delay4/1
  Delay3/1 -> Delay2/1, Inner Product/2(v)
  Delay5/1 -> Vector / Scalar Divide/2(y)
  Inner Product/2(validOut) -> Delay/1
  validIn/1 -> Delay1/1
  Vector / Scalar Divide/2(validOut) -> validOut/1
  Delay1/1 -> Inner Product/3(validIn)
  Delay2/1 -> Delay6/1
